simulink model "MotorXploer old"  (R2024b)
settings: Solver=FixedStepAuto  StartTime=0.0  StopTime=40  FixedStep=0.001  RelTol=1e-3
undefined symbols (not defined in the file or in its folder): Blocking, LF, Non
libraries: amg_usbconverter_n_connect_lib x3
settings Model: Creator=beamk  LastModifiedBy=pboon

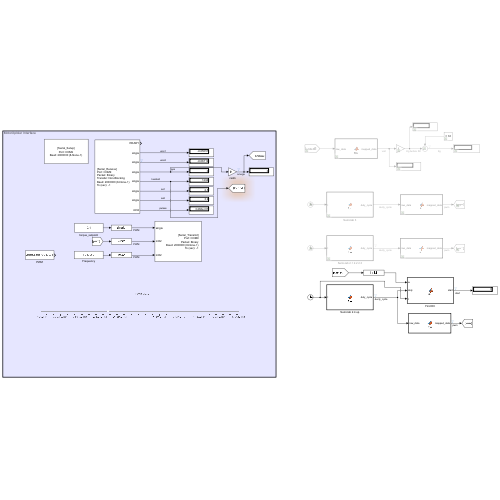
[thumbnail: Simulink's stored preview of the top-level diagram]
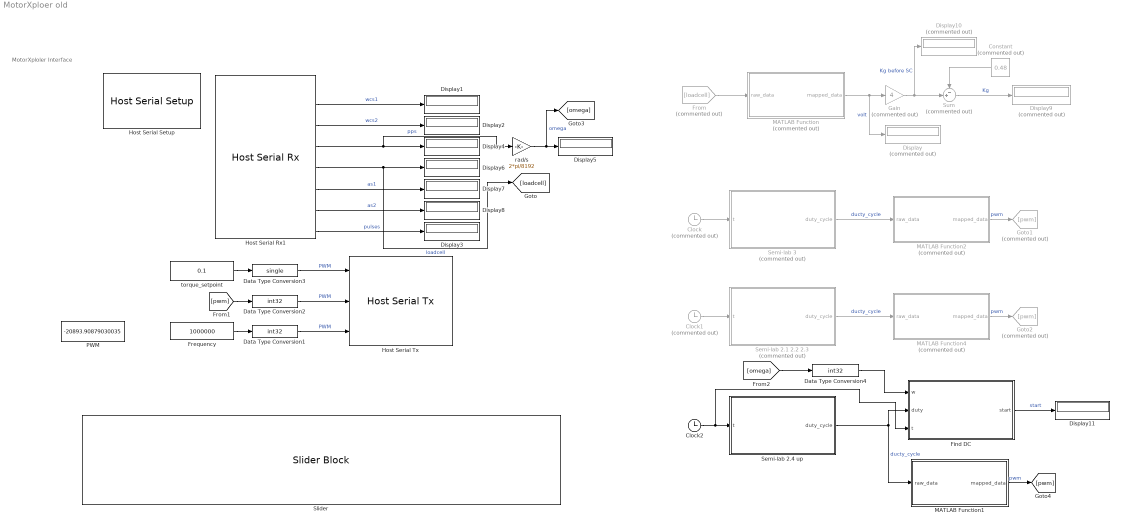
== system MotorXploer old ==
  note: MotorXploler Interface
  Clock : Clock  Commented=on
  Clock1 : Clock  Commented=on
  Clock2 : Clock
  Constant : Constant  Commented=on  Value=0.48
  Data Type Conversion1 : DataTypeConversion  OutDataTypeStr=int32  SaturateOnIntegerOverflow=off  RndMeth=Floor
  Data Type Conversion2 : DataTypeConversion  OutDataTypeStr=int32  SaturateOnIntegerOverflow=off  RndMeth=Floor
  Data Type Conversion3 : DataTypeConversion  OutDataTypeStr=single  SaturateOnIntegerOverflow=off  RndMeth=Floor
  Data Type Conversion4 : DataTypeConversion  OutDataTypeStr=int32  SaturateOnIntegerOverflow=off  RndMeth=Floor
  Display : Display  Commented=on
  Display{1..8,11} (9 alike) : Display
  Display10 : Display  Commented=on
  Display9 : Display  Commented=on
      settings: Format=bank
  Find DC : MATLAB Function  TreatAsAtomicUnit=on
  Frequency : Constant  Value=1000000
  From : From  Commented=on  GotoTag=loadcell
  Gain : Gain  Commented=on  Gain=4
  Goto1 : Goto  Commented=on  GotoTag=pwm
  Goto2 : Goto  Commented=on  GotoTag=pwm
  Host Serial Rx1 : amg_usbconverter_n_connect_lib/Host Serial Rx  conf=rx  port=<auto>  baudrate=2000000  databits=8  parity=None  stopbit=1  flowcontrol=None  transfer=Non-Blocking  timeout=5  packetmode=Binary  enableinitialvalues=off  initialvalues=[]  binheader='45'  binterminator='A'  porttype_double=0  porttype_single=6  porttype_int8=0  porttype_uint8=0  porttype_int16=0  porttype_uint16=0  porttype_int32=1  porttype_uint32=0  asciiformat='%f,%f,%d,%d'  rx_asciiterminator="LF (0x0A - \"\\n\")"  tx_asciiterminator="CRLF (0x0D 0x0A - \"\\r\\n\")"  sampletime=-1  enablecustomportlabel=off  cinputportlabel=0  coutputportlabel=A  portpinstr=0  blockid=HostSerialRx1  inputporttype=[]  inputportwidth=[]  inputportlabel={}  outputporttype=[3 1 1 1 1 1 1 6]  outputportwidth=[1 1 1 1 1 1 1 1]  outputportlabel={'READY','single','single','single','single','single','single','int32'}  compat=0  optionstring=[]  autoport='COM9'
  Host Serial Setup : amg_usbconverter_n_connect_lib/Host Serial Setup  conf=setup  port=<auto>  baudrate=2000000  databits=8  parity=None  stopbit=1  flowcontrol=None  transfer=Blocking  timeout=2  packetmode=Binary  initialvalues=[]  binheader='7E 7E'  binterminator='03 03'  porttype_double=0  porttype_single=1  porttype_int8=0  porttype_uint8=0  porttype_int16=0  porttype_uint16=0  porttype_int32=0  porttype_uint32=2  asciiformat='%d %u %x'  rx_asciiterminator="CRLF (0x0D 0x0A - \"\\r\\n\")"  tx_asciiterminator="CRLF (0x0D 0x0A - \"\\r\\n\")"  sampletime=-1  enablecustomportlabel=off  cinputportlabel=0  coutputportlabel=A  portpinstr=0  blockid=HostSerialSetup  inputporttype=[]  inputportwidth=[]  inputportlabel={}  outputporttype=[]  outputportwidth=[]  outputportlabel={}  compat=0  optionstring=[]  autoport='COM9'
  Host Serial Tx : amg_usbconverter_n_connect_lib/Host Serial Tx  conf=tx  port=<auto>  baudrate=2000000  databits=8  parity=None  stopbit=1  flowcontrol=None  transfer=Blocking  timeout=2  packetmode=Binary  initialvalues=[]  binheader='45'  binterminator='A'  porttype_double=0  porttype_single=1  porttype_int8=0  porttype_uint8=0  porttype_int16=0  porttype_uint16=0  porttype_int32=2  porttype_uint32=0  asciiformat='%d,%f'  rx_asciiterminator="CRLF (0x0D 0x0A - \"\\r\\n\")"  tx_asciiterminator="CRLF (0x0D 0x0A - \"\\r\\n\")"  sampletime=-1  enablecustomportlabel=off  cinputportlabel=0  coutputportlabel=A  portpinstr=0  blockid=HostSerialTx  inputporttype=[1 6 6]  inputportwidth=[1 1 1]  inputportlabel={'single','int32','int32'}  outputporttype=[]  outputportwidth=[]  outputportlabel={}  compat=0  optionstring=[]  autoport='COM9'
      settings: SourceProductName=aMG USB Converter N
  MATLAB Function : MATLAB Function  Commented=on  TreatAsAtomicUnit=on
  MATLAB Function1 : MATLAB Function  TreatAsAtomicUnit=on
  MATLAB Function2 : MATLAB Function  Commented=on  TreatAsAtomicUnit=on
  MATLAB Function4 : MATLAB Function  Commented=on  TreatAsAtomicUnit=on
  PWM : Constant  Value=-20893.90879030035
  Semi-lab 2.1 2.2 2.3 : MATLAB Function  Commented=on  TreatAsAtomicUnit=on
  Semi-lab 2.4 up : MATLAB Function  TreatAsAtomicUnit=on
  Semi-lab 3 : MATLAB Function  Commented=on  TreatAsAtomicUnit=on
  Slider : SliderBlock  ScaleMin=-65535  ScaleMax=65535
  Sum : Sum  Commented=on  Inputs=-+|
  rad/s : Gain  Gain=2*pi/8192
  torque_setpoint : Constant  Value=0.1
  wires:
  rad/s/1 -> [omega], Display5/1  "omega"
  Data Type Conversion1/1 -> Host Serial Tx/3  "PWM"
  Host Serial Rx1/8 -> Display3/1  "pulses"
  Host Serial Rx1/2 -> Display1/1  "wcs1"
  Frequency/1 -> Data Type Conversion1/1
  Data Type Conversion2/1 -> Host Serial Tx/2  "PWM"
  Host Serial Rx1/4 -> rad/s/1, Display4/1  "pps"
  Host Serial Rx1/3 -> Display2/1  "wcs2"
  Host Serial Rx1/5 -> [loadcell], Display6/1  "loadcell"
  Host Serial Rx1/6 -> Display7/1  "as1"
  Host Serial Rx1/7 -> Display8/1  "as2"
  Data Type Conversion3/1 -> Host Serial Tx/1  "PWM"
  torque_setpoint/1 -> Data Type Conversion3/1
  Sum/1 -> Display9/1  "Kg"
  Constant/1 -> Sum/1
  MATLAB Function/1(mapped_data) -> Display/1, Gain/1  "volt"
  Gain/1 -> Display10/1, Sum/2  "Kg before SC"
  From/1 -> MATLAB Function/1(raw_data)
  Clock/1 -> Semi-lab 3/1(t)
  Semi-lab 3/1(duty_cycle) -> MATLAB Function2/1(raw_data)  "ducty_cycle"
  MATLAB Function2/1(mapped_data) -> Goto1/1  "pwm"
  Semi-lab 2.1 2.2 2.3/1(duty_cycle) -> MATLAB Function4/1(raw_data)  "ducty_cycle"
  MATLAB Function4/1(mapped_data) -> Goto2/1  "pwm"
  Clock1/1 -> Semi-lab 2.1 2.2 2.3/1(t)
  [pwm] -> Data Type Conversion2/1
  Clock2/1 -> Find DC/3(t), Semi-lab 2.4 up/1(t)
  Semi-lab 2.4 up/1(duty_cycle) -> Find DC/2(duty), MATLAB Function1/1(raw_data)  "ducty_cycle"
  MATLAB Function1/1(mapped_data) -> [pwm]  "pwm"
  Find DC/1(start) -> Display11/1  "start"
  [omega] -> Data Type Conversion4/1
  Data Type Conversion4/1 -> Find DC/1(w)

== matlab function MotorXploer old/MATLAB Function ==
  data: raw_data input; mapped_data output
function mapped_data = fcn(raw_data)

in_min = 0.0;
out_min = 0.0;
in_max = 4095.0;
out_max = 3.3;

mapped_data =  (double(raw_data) - in_min) * (out_max - out_min) / (in_max - in_min) + out_min;

== matlab function MotorXploer old/MATLAB Function2 ==
  data: raw_data input; mapped_data output
function mapped_data = fcn(raw_data)

in_min = 0.0;
out_min = 0.0;
in_max = 100.0;
out_max = 65535.0;

mapped_data =  (double(raw_data) - in_min) * (out_max - out_min) / (in_max - in_min) + out_min;

== matlab function MotorXploer old/Semi-lab 2.1 2.2 2.3 ==
  data: t input; duty_cycle output
function duty_cycle = fcn(t)

duty_cycle = 5*t;

== matlab function MotorXploer old/MATLAB Function4 ==
  data: raw_data input; mapped_data output
function mapped_data = fcn(raw_data)

in_min = 0.0;
out_min = 0.0;
in_max = 100.0;
out_max = 65535.0;

mapped_data =  (double(raw_data) - in_min) * (out_max - out_min) / (in_max - in_min) + out_min;

== matlab function MotorXploer old/Find DC ==
  data: w input; start output; duty input; t input
function start = fcn(w, duty, t)
persistent firstStartDuty firststopDuty

if isempty(firstStartDuty)
    firstStartDuty = NaN; 
end

if isempty(firststopDuty)
    firststopDuty = NaN; 
end

if w > 0.0 && isnan(firstStartDuty) && duty >= 1 && t <= 20
    firstStartDuty = duty;
    start = firstStartDuty;
elseif w == 0.0 && isnan(firststopDuty) && t > 20
    firststopDuty = duty;
    start = firststopDuty;
else
    start = 0.0;
end

== matlab function MotorXploer old/Semi-lab 2.4 up ==
  data: t input; duty_cycle output
function duty_cycle = fcn(t)
if t <= 20
    duty_cycle = 5 * t;
elseif t <= 40
    duty_cycle = 100 - (5 * (t - 20));
else
    duty_cycle = 0;
end

== matlab function MotorXploer old/MATLAB Function1 ==
  data: raw_data input; mapped_data output
function mapped_data = fcn(raw_data)

in_min = 0.0;
out_min = 0.0;
in_max = 100.0;
out_max = 65535.0;

mapped_data =  (double(raw_data) - in_min) * (out_max - out_min) / (in_max - in_min) + out_min;

== matlab function MotorXploer old/Semi-lab 3 ==
  data: t input; duty_cycle output
function duty_cycle = fcn(t)
duty_cycle_values = [50, 60, 70, 80, 90, 100, 90, 80, 70, 60, 50, 40, 30, 20, 10, 0, 10, 20, 30, 40, 50];

step_duration = 2.5; 

cycle_duration = numel(duty_cycle_values) * step_duration;

t_mod = mod(t, cycle_duration);

step_index = floor(t_mod / step_duration) + 1;

duty_cycle = duty_cycle_values(step_index);
